simulink model "Q3sim"  (R2018a)
settings: Solver=VariableStepAuto  StartTime=0.0  StopTime=10.0  RelTol=1e-3
values from neighbouring files (symbols this model uses):
  A = [0 1 0 0 ;0 -2.2626 -0.3962 0.0082; 0 0 0 1;0 3.5649 16.0655 -0.3324]    [Q1.m]    (also in Q2.m; Q3.m; Q4.m)
  B = [0; 0.2263; 0; -0.3565]    [Q1.m]    (also in Q2.m; Q3.m; Q4.m)
  C = eye(4,4)    [Q1.m]    (also in Q2.m; Q3.m; Q4.m = [1 0 0 0])
  D = [0 0 0 0]'    [Q1.m]    (also in Q2.m; Q3.m; Q4.m = 0)
  K = acker(Abar,Bbar,[-1 -2 -3 -4 -5])    [Q2.m]    (also in Q3.m = acker(A,B,[-1 -2 -3 -4]); Q4.m = acker(A,B,[-1 -2 -3 -4]))
libraries: peLuenbergerObserver x1
settings Model: Creator=Siavash  LastModifiedBy=Siavash

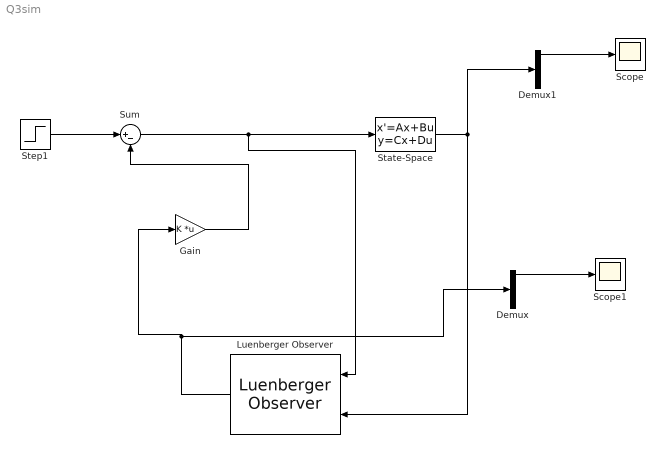
== system Q3sim ==
  Demux : Demux
  Demux1 : Demux
  Gain : Gain  Gain=K  Multiplication=Matrix(K*u)
  Luenberger Observer : peLuenbergerObserver/Luenberger Observer  StateSpaceType=Continuous-time  Ad=A  Bd=B  Cd=C  Dd=D  A=A  B=B  C=C  D=D  ObserverDesign=Desired eigenvalues  Ld=1  DesiredEigenvalues=[-1 -2 -3 -4]  x0=[0 0 0 0]  Tsd=0.1  Ts=0.01
  Scope : Scope
  Scope1 : Scope
  State-Space : StateSpace  A=A  B=B  C=C  D=D  InitialCondition=0
  Step1 : Step  Time=0  SampleTime=0
  Sum : Sum  Inputs=|+-
  wires:
  Sum/1 -> Luenberger Observer/1, State-Space/1
  State-Space/1 -> Demux1/1, Luenberger Observer/2
  Step1/1 -> Sum/1
  Demux/1 -> Scope1/1
  Luenberger Observer/1 -> Demux/1, Gain/1
  Gain/1 -> Sum/2
  Demux1/1 -> Scope/1
